simulink model "sampleModel1904_2_sub_sub"  (R2023a)
settings: Solver=VariableStepAuto  StartTime=0.0  StopTime=10.0  RelTol=1e-3
libraries: hdlsllib x3, simulink x1
settings Model: Creator=user1  LastModifiedBy=user1
settings OptimizationCC: BlockReduction=off  ConditionallyExecuteInputs=off

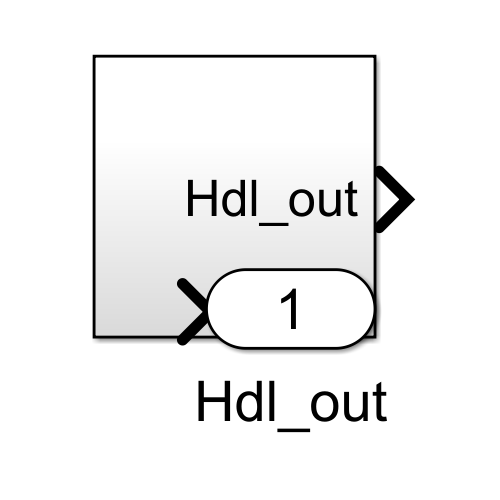
[thumbnail: Simulink's stored preview of the top-level diagram]
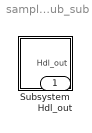
== system sampleModel1904_2_sub_sub ==
  Subsystem : Subsystem
  Hdl_out : Outport  OutDataTypeStr=uint8

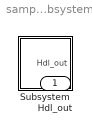
== system sampleModel1904_2_sub_sub/Subsystem ==
  Subsystem : Subsystem
  Hdl_out : Outport  OutDataTypeStr=uint8

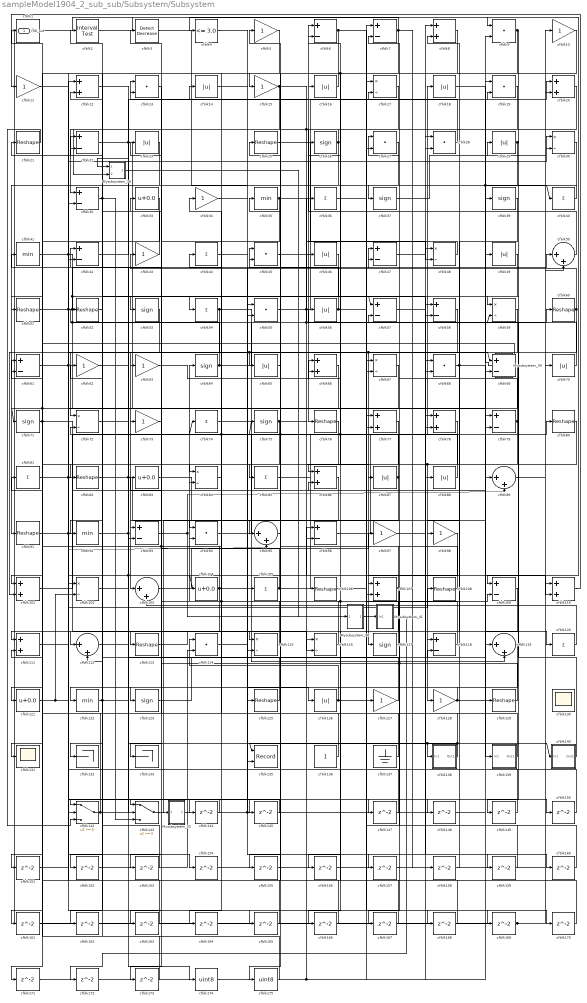
== system sampleModel1904_2_sub_sub/Subsystem/Subsystem ==
  Mysubsystem_33 : Subsystem  TreatAsAtomicUnit=on  RTWFcnName=Mysubsystem_33
      settings: RTWFcnNameOpts=User specified  RTWFileNameOpts=Use function name
  Mysubsystem_36 : Subsystem  TreatAsAtomicUnit=on  RTWFcnName=Mysubsystem_36
      settings: RTWFcnNameOpts=User specified  RTWFileNameOpts=Use function name
  Mysubsystem_38 : Subsystem  TreatAsAtomicUnit=on  RTWFcnName=Mysubsystem_38
      settings: RTWFcnNameOpts=User specified  RTWFileNameOpts=Use function name
  Mysubsystem_39 : Subsystem  TreatAsAtomicUnit=on  RTWFcnName=Mysubsystem_39
      settings: RTWFcnNameOpts=User specified  RTWFileNameOpts=Use function name
  Mysubsystem_41 : Subsystem  TreatAsAtomicUnit=on  RTWFcnName=Mysubsystem_41
      settings: RTWFcnNameOpts=User specified  RTWFileNameOpts=Use function name
  cfblk1 : hdlsllib/Logic and Bit Operations/Compare To Zero  relop=<=  OutDataTypeStr=uint8
  cfblk{5,10..11,15,34,43,62..63,73,97..98,127..128} (13 alike) : Gain  OutDataTypeStr=uint8
  cfblk{8,12,20,66,77..78,86,101,107,110..111} (11 alike) : Sum  OutDataTypeStr=uint8
  cfblk{17,30,48,59,67,72,84,102,115..116} (10 alike) : Product  Inputs=*/  OutDataTypeStr=uint8  RndMeth=Zero  SaturateOnIntegerOverflow=on
  cfblk{50,89,95,103,112,119} (6 alike) : Sum  Inputs=|++  OutDataTypeStr=uint8
  cfblk{33,83,104,121} (4 alike) : Bias  Bias=0.0  SaturateOnIntegerOverflow=off
  cfblk{36,40,44,54,74,81,85,105,120} (9 alike) : Sum  Inputs=+  OutDataTypeStr=uint8
  cfblk{21,25,51..52,60,76,80,82,91,106,108,113,125,129} (14 alike) : Reshape
  cfblk{6..7,22,32,42,47,57..58,61,69,79,93,96,109,118} (15 alike) : Sum  Inputs=+-  OutDataTypeStr=uint8
  cfblk{9,13,19,27..28,45,55,68,94,114} (10 alike) : DotProduct  OutDataTypeStr=uint8
  cfblk{26,37,39,53,64,71,75,117,123} (9 alike) : Signum
  cfblk{35,41,92,122} (4 alike) : MinMax  OutDataTypeStr=uint8
  cfblk{14,16,18,23,29,46,49,56,65,70,87..88,126} (13 alike) : Abs  OutDataTypeStr=uint8  SaturateOnIntegerOverflow=off
  cfblk130 : Scope
      settings: Floating=on
  cfblk131 : Scope
  cfblk132 : Terminator
  cfblk133 : Terminator
  cfblk135 : Record  FileSettingsInternal="{\"entries\":[{\"content\":{\"excelSettings\":{\"content\":{},\"type\":\"Streamout.ExcelSettings\"}},\"type\":\"Streamout.FileSettingStorage\",\"uuid\":\"\"}],\"packageUris\":[\"http:\\/\\/schema.mathworks.com\\/mf0\\/streamout_blocks\\/R2020a\"],\"version\":\"1.0\"}"  Layout=[1 1]  SignalsInternal="{\"entries\":[{\"content\":{\"signals\":[{\"content\":{\"blockPath\":[],\"dimensions\":[1],\"domain\":\"\",\"lineColor\":\"#a2142f\",\"plots\":[1],\"port\":1,\"signalID\":50152,\"signalName\":\"cfblk138\"},\"type\":\"RecordBlkView.Signal\",\"uuid\":\"\"},{\"content\":{\"blockPath\":[],\"dimensions\":[1],\"domain\":\"\",\"lineColor\":\"#139fff\",\"plots\":[1],\"port\":2,\"signalID\":50155,\"signalName\":\"cfblk92\"},\"type\":\"RecordBlkView.Signal\",\"uuid\":\"\"}]},\"type\":\"RecordBlkView.InputSignals\",\"uuid\":\"\"}],\"packageUris\":[\"http:\\/\\/schema.mathworks.com\\/mf0\\/streamout_blocks\\/R2020a\"],\"version\":\"1.0\"}"  VisualizationBindings="{\"xyplotplugin\":{\"info\":[{\"series\":[{\"bindingParametersList\":[{\"parameter\":\"X-Axis\",\"signalID\":50152,\"signalName\":\"cfblk138\"},{\"parameter\":\"Y-Axis\",\"signalID\":50155,\"signalName\":\"cfblk92\"}],\"seriesID\":31541}],\"subplotID\":1}]}}"  CompatibilityTag=XY  st=-1
  cfblk136 : Constant  OutDataTypeStr=uint8  SampleTime=-1
  cfblk137 : Ground
  cfblk138 : Subsystem
      settings: LibrarySourceBlock=|
      | hdlsllib/Ports &
      | Subsystems/Subsystem
  cfblk139 : Subsystem
      settings: LibrarySourceBlock=|
      | hdlsllib/Ports &
      | Subsystems/Subsystem
  cfblk140 : Subsystem
      settings: LibrarySourceBlock=|
      | hdlsllib/Ports &
      | Subsystems/Subsystem
  cfblk142 : Switch  OutDataTypeStr=uint8  SaturateOnIntegerOverflow=off  InputSameDT=off
  cfblk143 : Switch  OutDataTypeStr=uint8  SaturateOnIntegerOverflow=off  InputSameDT=off
  cfblk{144..145,147..173} (29 alike) : Delay  SampleTime=1
  cfblk174 : DataTypeConversion  OutDataTypeStr=uint8  SaturateOnIntegerOverflow=off  RndMeth=Floor
  cfblk175 : DataTypeConversion  OutDataTypeStr=uint8  SaturateOnIntegerOverflow=off  RndMeth=Floor
  cfblk2 : hdlsllib/Logic and Bit Operations/Interval Test  IntervalClosedRight=on  uplimit=0.5  IntervalClosedLeft=on  lowlimit=-0.5  OutDataTypeStr=uint8
  cfblk3 : simulink/Logic and Bit Operations/Detect Decrease  vinit=0.0  OutDataTypeStr=uint8
      settings: LibrarySourceBlock=|
      | hdlsllib/Logic and Bit
      | Operations/Detect
      | Decrease
  cfblk4 : hdlsllib/Logic and Bit Operations/Compare To Constant  relop=<=  const=3.0  OutDataTypeStr=uint8
  Hdl_out : Outport  OutDataTypeStr=uint8
  wires:
  Mysubsystem_39/1(Out1) -> cfblk151/1
  Mysubsystem_38/1(Out1) -> cfblk172/1
  Mysubsystem_36/1(Out1) -> Mysubsystem_38/1(In1)
  Mysubsystem_33/1(Out1) -> cfblk28/1
  cfblk86/1 -> Mysubsystem_33/1(In1)
  cfblk175/1 -> cfblk62/1
  cfblk174/1 -> cfblk89/1, cfblk106/1
  cfblk173/1 -> cfblk1/1
  cfblk172/1 -> cfblk68/2
  cfblk171/1 -> cfblk27/2
  cfblk170/1 -> cfblk102/1
  cfblk169/1 -> cfblk20/2, Hdl_out/1
  cfblk168/1 -> cfblk111/2
  cfblk167/1 -> cfblk6/2
  cfblk166/1 -> cfblk45/2
  cfblk165/1 -> cfblk22/2
  cfblk164/1 -> cfblk110/1
  cfblk163/1 -> cfblk112/2
  cfblk162/1 -> cfblk96/1
  cfblk49/1 -> cfblk162/1
  cfblk161/1 -> cfblk116/1
  cfblk66/1 -> cfblk161/1
  cfblk160/1 -> cfblk77/1
  cfblk57/1 -> cfblk160/1
  cfblk159/1 -> cfblk17/2
  cfblk44/1 -> cfblk159/1
  cfblk158/1 -> cfblk8/2
  cfblk157/1 -> cfblk79/1
  cfblk4/1 -> cfblk157/1
  cfblk156/1 -> cfblk19/1
  cfblk119/1 -> cfblk156/1
  cfblk155/1 -> cfblk50/2
  cfblk65/1 -> cfblk155/1
  cfblk154/1 -> cfblk58/1
  cfblk153/1 -> cfblk72/2
  cfblk73/1 -> cfblk153/1
  cfblk152/1 -> cfblk114/2
  cfblk151/1 -> cfblk32/2
  cfblk150/1 -> cfblk55/1
  cfblk97/1 -> cfblk150/1
  cfblk149/1 -> cfblk78/1
  cfblk148/1 -> cfblk9/2
  cfblk106/1 -> cfblk148/1
  cfblk147/1 -> cfblk12/1
  cfblk145/1 -> cfblk143/1
  cfblk95/1 -> cfblk145/1
  cfblk144/1 -> cfblk142/2
  cfblk84/1 -> cfblk144/1
  cfblk15/1 -> cfblk48/2, cfblk152/1
  cfblk70/1 -> cfblk27/1
  cfblk101/1 -> cfblk69/2
  cfblk61/1 -> cfblk69/1, cfblk65/1, cfblk154/1
  cfblk92/1 -> cfblk84/2, cfblk135/2
  cfblk68/1 -> cfblk118/1, cfblk120/1
  cfblk25/1 -> cfblk67/1
  cfblk47/1 -> cfblk20/1
  cfblk23/1 -> cfblk111/1
  cfblk21/1 -> cfblk142/3
  cfblk11/1 -> cfblk78/2
  cfblk39/1 -> cfblk98/1
  cfblk72/1 -> cfblk104/1, cfblk170/1
  cfblk33/1 -> cfblk101/1, cfblk71/1
  cfblk122/1 -> cfblk22/1, cfblk118/2
  cfblk28/1 -> cfblk14/1
  cfblk83/1 -> cfblk139/1(In1)
  cfblk98/1 -> cfblk107/1
  cfblk19/1 -> cfblk96/2, cfblk173/1
  cfblk6/1 -> cfblk58/2, cfblk175/1
  cfblk43/1 -> cfblk12/2
  cfblk136/1 -> cfblk94/2
  cfblk77/1 -> cfblk121/1
  cfblk64/1 -> cfblk28/2, cfblk36/1, cfblk52/1
  cfblk110/1 -> cfblk11/1
  cfblk37/1 -> cfblk29/1
  cfblk75/1 -> cfblk110/2, cfblk92/1
  cfblk80/1 -> cfblk82/1
  cfblk111/1 -> cfblk108/1
  cfblk143/1 -> cfblk55/2, cfblk39/1
  cfblk52/1 -> cfblk142/1
  cfblk18/1 -> Mysubsystem_39/1(In1), cfblk40/1
  cfblk48/1 -> cfblk46/1
  cfblk34/1 -> cfblk126/1
  cfblk12/1 -> cfblk116/2
  cfblk138/1(Out1) -> cfblk13/2, cfblk135/1
  cfblk120/1 -> cfblk103/2
  cfblk89/1 -> cfblk10/1
  cfblk81/1 -> cfblk48/1, cfblk95/2
  cfblk45/1 -> cfblk8/1
  cfblk10/1 -> cfblk95/1
  cfblk36/1 -> cfblk77/2
  cfblk7/1 -> cfblk4/1, cfblk42/2, cfblk158/1
  cfblk30/1 -> cfblk93/2
  cfblk63/1 -> cfblk66/2
  cfblk103/1 -> cfblk97/1
  cfblk35/1 -> cfblk87/1, cfblk163/1
  cfblk88/1 -> cfblk66/1, cfblk2/1
  cfblk121/1 -> cfblk102/2, cfblk147/1
  cfblk125/1 -> cfblk21/1
  cfblk96/1 -> cfblk68/1
  cfblk116/1 -> cfblk23/1
  cfblk140/1(Out1) -> cfblk56/1
  cfblk17/1 -> cfblk32/1
  cfblk79/1 -> cfblk85/1, cfblk57/2
  cfblk13/1 -> cfblk133/1
  cfblk104/1 -> cfblk138/1(In1), cfblk140/1(In1), cfblk3/1, cfblk61/2, cfblk131/1
  cfblk129/1 -> cfblk33/1, cfblk7/2
  cfblk54/1 -> cfblk129/1, cfblk63/1
  cfblk123/1 -> cfblk49/1
  cfblk71/1 -> cfblk115/2, cfblk171/1
  cfblk55/1 -> cfblk19/2, cfblk47/2
  cfblk139/1(Out1) -> cfblk42/1
  cfblk14/1 -> cfblk125/1
  cfblk137/1 -> cfblk61/1
  cfblk109/1 -> cfblk123/1
  cfblk107/1 -> cfblk35/1, cfblk166/1, cfblk167/1
  cfblk93/1 -> cfblk89/2, Mysubsystem_41/1(In1)
  cfblk5/1 -> cfblk94/1
  cfblk8/1 -> cfblk51/1
  cfblk91/1 -> cfblk70/1, cfblk30/1
  cfblk94/1 -> cfblk80/1
  cfblk32/1 -> cfblk132/1, cfblk143/3
  cfblk114/1 -> cfblk47/1
  cfblk85/1 -> cfblk17/1
  cfblk82/1 -> cfblk127/1, cfblk165/1
  cfblk87/1 -> cfblk5/1, cfblk164/1
  cfblk29/1 -> cfblk53/1, cfblk149/1
  cfblk112/1 -> cfblk60/1
  cfblk128/1 -> cfblk122/1, cfblk30/2
  cfblk62/1 -> cfblk174/1
  cfblk3/1 -> cfblk105/1
  cfblk41/1 -> cfblk57/1, cfblk88/1, cfblk107/2
  cfblk142/1 -> cfblk81/1, cfblk86/2
  cfblk56/1 -> cfblk45/1, cfblk169/1
  cfblk127/1 -> cfblk25/1
  cfblk1/1 -> cfblk9/1
  cfblk9/1 -> cfblk112/1, cfblk86/1, cfblk59/1
  cfblk108/1 -> cfblk13/1, cfblk75/1
  cfblk67/1 -> cfblk93/1
  cfblk42/1 -> cfblk16/1
  cfblk50/1 -> cfblk6/1
  cfblk105/1 -> cfblk18/1, cfblk83/1
  cfblk102/1 -> cfblk50/1
  cfblk76/1 -> cfblk113/1
  cfblk69/1 -> cfblk73/1
  cfblk46/1 -> cfblk84/1
  cfblk78/1 -> cfblk128/1, cfblk143/2
  cfblk118/1 -> cfblk34/1, cfblk26/1
  cfblk2/1 -> cfblk109/1
  cfblk113/1 -> cfblk115/1
  cfblk126/1 -> cfblk114/1, cfblk109/2
  cfblk27/1 -> cfblk54/1
  cfblk59/1 -> cfblk117/1, cfblk67/2
  cfblk74/1 -> cfblk119/2
  cfblk117/1 -> cfblk44/1, cfblk74/1, cfblk41/1
  cfblk60/1 -> cfblk43/1, cfblk101/2
  cfblk20/1 -> cfblk76/1
  cfblk51/1 -> cfblk119/1, cfblk59/2, cfblk7/1, cfblk168/1
  cfblk58/1 -> cfblk72/1
  cfblk115/1 -> cfblk64/1
  cfblk22/1 -> Mysubsystem_36/1(In1), cfblk79/2
  cfblk16/1 -> cfblk15/1
  cfblk40/1 -> cfblk37/1
  cfblk26/1 -> Mysubsystem_36/2(In2), cfblk91/1
  cfblk53/1 -> cfblk103/1

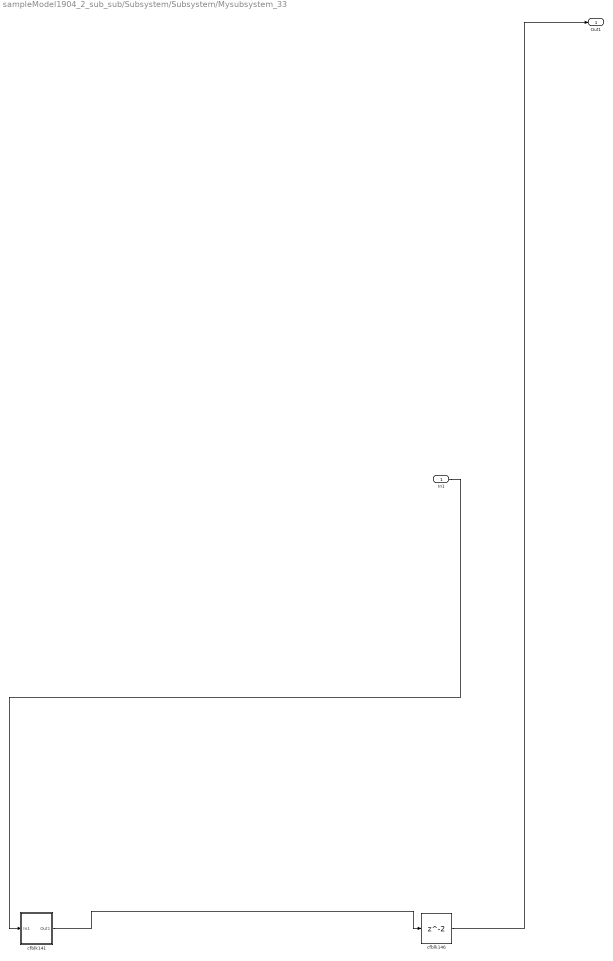
== system sampleModel1904_2_sub_sub/Subsystem/Subsystem/Mysubsystem_33 ==
  In1 : Inport
  cfblk141 : Subsystem
      settings: LibrarySourceBlock=|
      | hdlsllib/Ports &
      | Subsystems/Subsystem
  cfblk146 : Delay  SampleTime=1
  Out1 : Outport
  wires:
  cfblk141/1(Out1) -> cfblk146/1
  cfblk146/1 -> Out1/1
  In1/1 -> cfblk141/1(In1)

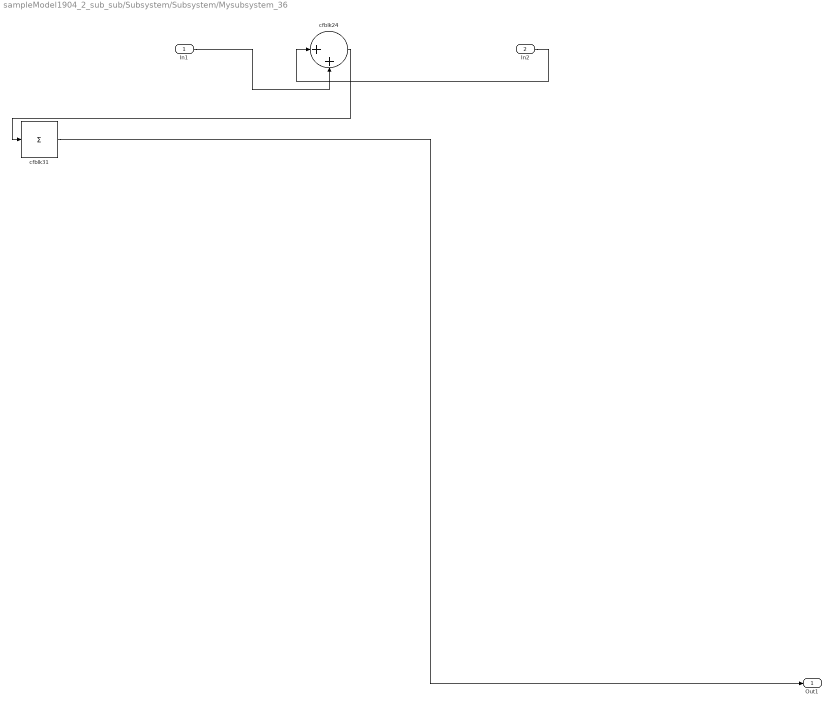
== system sampleModel1904_2_sub_sub/Subsystem/Subsystem/Mysubsystem_36 ==
  In1 : Inport
  In2 : Inport  Port=2
  cfblk24 : Sum  Inputs=|++
  cfblk31 : Sum  Inputs=+
  Out1 : Outport
  wires:
  cfblk31/1 -> Out1/1
  In2/1 -> cfblk24/1
  cfblk24/1 -> cfblk31/1
  In1/1 -> cfblk24/2

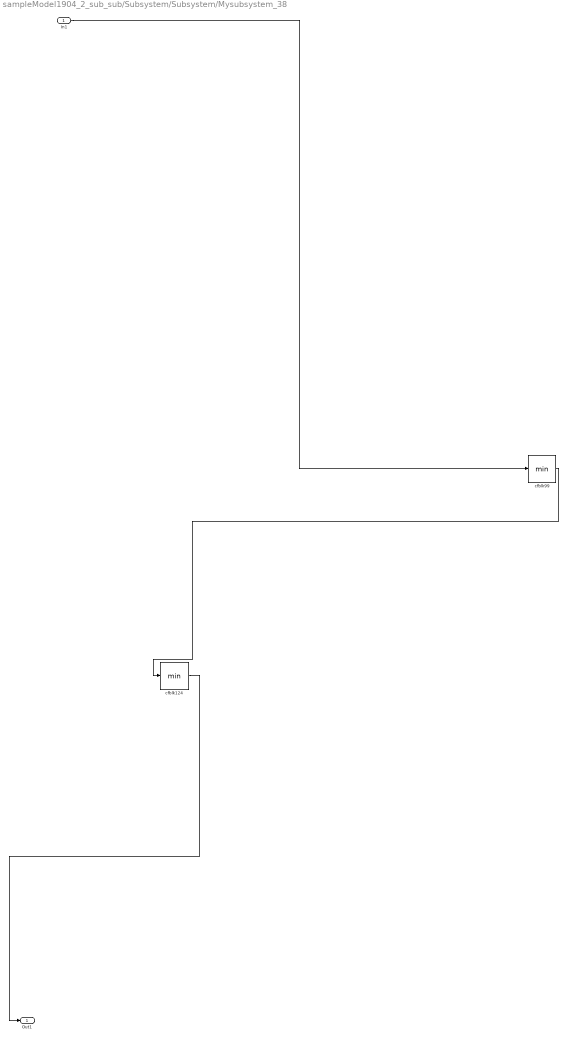
== system sampleModel1904_2_sub_sub/Subsystem/Subsystem/Mysubsystem_38 ==
  In1 : Inport
  cfblk124 : MinMax
  cfblk99 : MinMax
  Out1 : Outport
  wires:
  cfblk99/1 -> cfblk124/1
  In1/1 -> cfblk99/1
  cfblk124/1 -> Out1/1

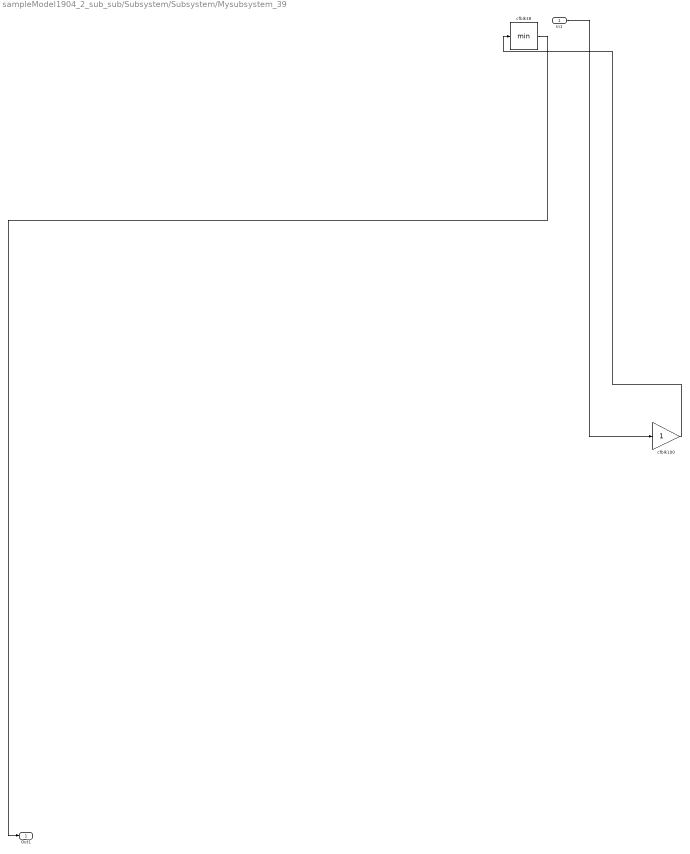
== system sampleModel1904_2_sub_sub/Subsystem/Subsystem/Mysubsystem_39 ==
  In1 : Inport
  cfblk100 : Gain
  cfblk38 : MinMax
  Out1 : Outport
  wires:
  In1/1 -> cfblk100/1
  cfblk38/1 -> Out1/1
  cfblk100/1 -> cfblk38/1

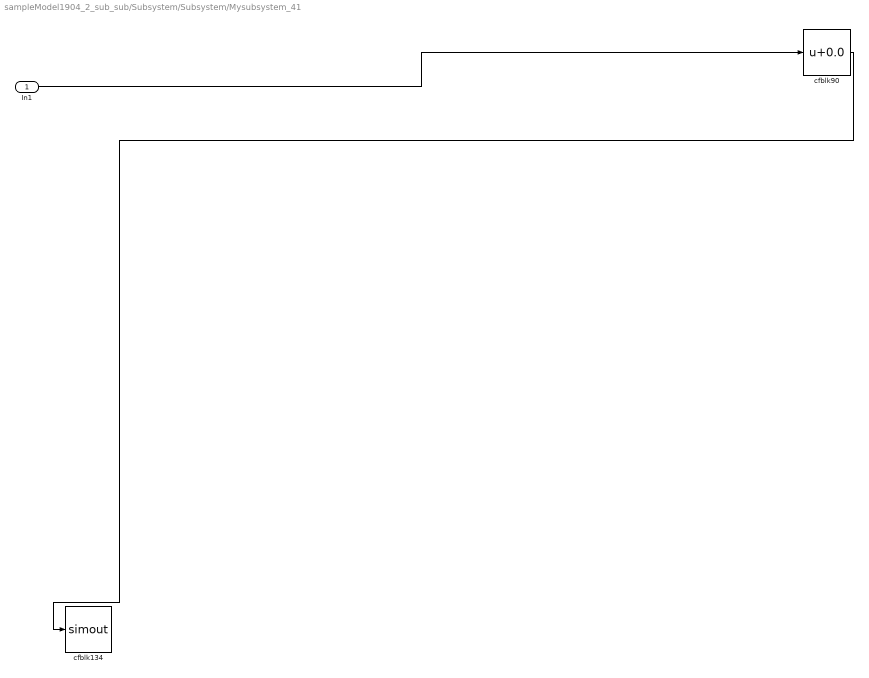
== system sampleModel1904_2_sub_sub/Subsystem/Subsystem/Mysubsystem_41 ==
  In1 : Inport
  cfblk134 : ToWorkspace  VariableName=simout  SaveFormat=Timeseries  SampleTime=-1
  cfblk90 : Bias  Bias=0.0  SaturateOnIntegerOverflow=off
  wires:
  In1/1 -> cfblk90/1
  cfblk90/1 -> cfblk134/1

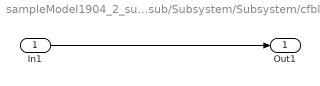
== system sampleModel1904_2_sub_sub/Subsystem/Subsystem/cfblk138 ==
  In1 : Inport
  Out1 : Outport
  wires:
  In1/1 -> Out1/1

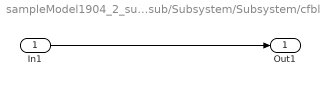
== system sampleModel1904_2_sub_sub/Subsystem/Subsystem/cfblk139 ==
  In1 : Inport
  Out1 : Outport
  wires:
  In1/1 -> Out1/1

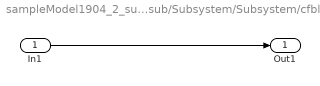
== system sampleModel1904_2_sub_sub/Subsystem/Subsystem/cfblk140 ==
  In1 : Inport
  Out1 : Outport
  wires:
  In1/1 -> Out1/1

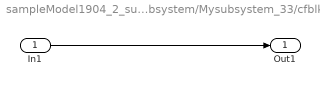
== system sampleModel1904_2_sub_sub/Subsystem/Subsystem/Mysubsystem_33/cfblk141 ==
  In1 : Inport
  Out1 : Outport
  wires:
  In1/1 -> Out1/1
